simulink model "gm_ThreeSines_DrSaher"  (R2018a)
settings: Solver=FixedStepDiscrete  StartTime=0.0  StopTime=0.01  RelTol=1e-3
InitFcn:
  | ST = 2e-8
  | Ts = 2e-8
libraries: hdlmdlgenlib x97, hdlsllib x13, simulink x7, powerlib x1
(part 1 of 3)
settings Model: SimulationMode=accelerator  Creator=aaala  LastModifiedBy=aaala
settings OptimizationCC: BlockReduction=off  ConditionallyExecuteInputs=off  DefaultParameterBehavior=Inlined
settings DebuggingCC: AlgebraicLoopMsg=error  InheritedTsInSrcMsg=none  SingleTaskRateTransMsg=error
settings HardwareCC: ProdBitPerPointer=32  ProdBitPerSizeT=32  ProdBitPerPtrDiffT=32  ProdLargestAtomicFloat=None  ProdIntDivRoundTo=Undefined  ProdEndianess=Unspecified  ProdWordSize=32  ProdHWDeviceType=ASIC/FPGA->ASIC/FPGA  TargetBitPerPointer=64  TargetBitPerSizeT=64  TargetBitPerPtrDiffT=64  TargetLongLongMode=on  TargetIntDivRoundTo=Zero  TargetEndianess=LittleEndian  TargetWordSize=64  TargetHWDeviceType=Custom Processor->MATLAB Host Computer  ProdEqTarget=off

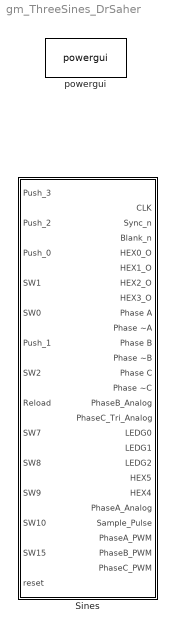
== system gm_ThreeSines_DrSaher ==
  "Sines " : Subsystem
  powergui : powerlib/powergui  Priority=1  SimulationMode=Discrete  SampleTime=ST  frequency=60  Iterations=50  frequencyindice=60  Pbase=100e6  ErrMax=1e-4  UnitsV=kV  UnitsW=MW  buscounter=0  FunctionMessages=off  echomessages=off  EnableUseOfTLC=off  CurrentSourceSwitches=off  DisableSnubberDevices=off  DisableRonSwitches=off  DisableVfSwitches=off  DisplayEquations=off  SolverType=Tustin/Backward Euler (TBE)  Interpol=off  ExternalGateDelay=off  methode=off  Ts=100  x0status=blocks  SPID=on  SwTol=0  HookPort=off  RestoreLinks=warning  ResistiveCurrentMeasurement=off  Frange=[0:2:500]  Ylog=off  Xlog=on  ShowGrid=off  save=off  variable=ZData  structure=0  ZoomFFT=off  StartTime=0.0  cycles=1  DisplayStyle=1  fundamental=60  FreqAxis=off  MaxFrequency=1000  frequencyindicesteady=1  RmsSteady=1  display=off

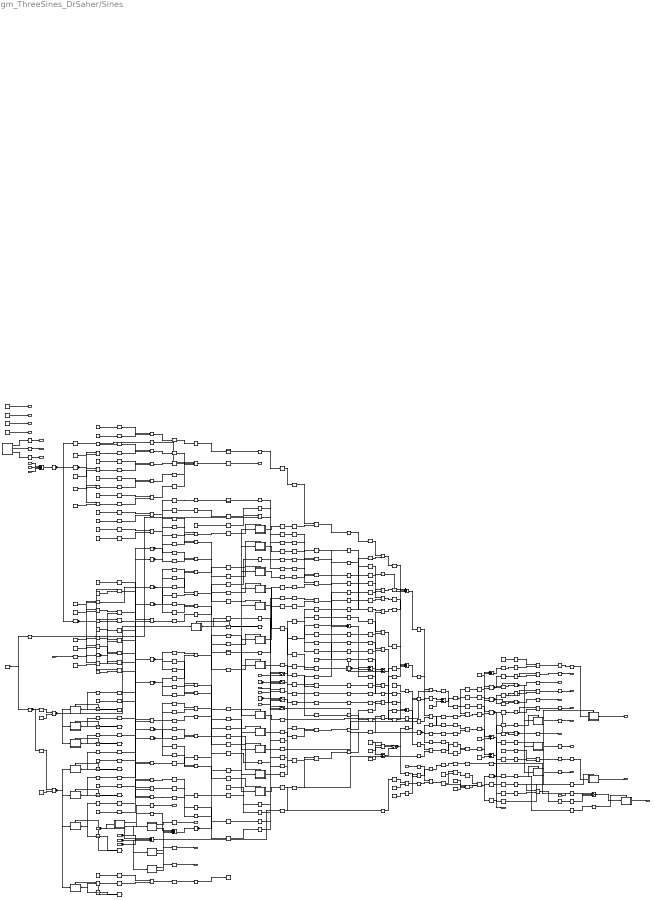
== system gm_ThreeSines_DrSaher/Sines  ==
  note: 999945
  "Push_3 " : Inport  OutDataTypeStr=boolean  PortDimensions=1  SampleTime=2e-08
  Push_2 : Inport  Port=2  OutDataTypeStr=boolean  PortDimensions=1  SampleTime=2e-08
  Push_0 : Inport  Port=3  OutDataTypeStr=boolean  PortDimensions=1  SampleTime=2e-08
  SW1 : Inport  Port=4  OutDataTypeStr=boolean  PortDimensions=1  SampleTime=2e-08
  SW0 : Inport  Port=5  OutDataTypeStr=boolean  PortDimensions=1  SampleTime=2e-08
  Push_1 : Inport  Port=6  OutDataTypeStr=boolean  PortDimensions=1  SampleTime=2e-08
  "SW2 " : Inport  Port=7  OutDataTypeStr=boolean  PortDimensions=1  SampleTime=2e-08
  Reload : Inport  Port=8  OutDataTypeStr=boolean  PortDimensions=1  SampleTime=2e-08
  "SW7 " : Inport  Port=9  OutDataTypeStr=boolean  PortDimensions=1  SampleTime=2e-08
  SW8 : Inport  Port=10  OutDataTypeStr=boolean  PortDimensions=1  SampleTime=2e-08
  SW9 : Inport  Port=11  OutDataTypeStr=boolean  PortDimensions=1  SampleTime=2e-08
  SW10 : Inport  Port=12  OutDataTypeStr=boolean  PortDimensions=1  SampleTime=2e-08
  SW15 : Inport  Port=13  OutDataTypeStr=boolean  PortDimensions=1  SampleTime=2e-08
  reset : Inport  Port=14  OutDataTypeStr=boolean  PortDimensions=1  SampleTime=2e-08
  Constant : Constant  Value=fi(0,0,32,0,'hex','00001387')  OutDataTypeStr=uint32  SampleTime=-1
  Constant10 : Constant  Value=fi(0,1,16,11,'hex','6000')  OutDataTypeStr=fixdt(1, 16, 11)  SampleTime=-1
  Constant11 : Constant  Value=fi(0,1,16,13,'hex','2000')  OutDataTypeStr=fixdt(1, 16, 13)  SampleTime=-1
  Constant12 : Constant  Value=fi(0,1,16,3,'hex','4d20')  OutDataTypeStr=fixdt(1, 16, 3)  SampleTime=-1
  Constant13 : Constant  Value=fi(0,0,20,0,'hex','51603')  OutDataTypeStr=fixdt(0, 20, 0)  SampleTime=-1
  Constant14 : Constant  Value=fi(0,1,16,6,'hex','6540')  OutDataTypeStr=fixdt(1, 16, 6)  SampleTime=-1
  Constant15 : Constant  Value=fi(0,0,3,0,'hex','4')  OutDataTypeStr=fixdt(0, 3, 0)  SampleTime=-1
  Constant17 : Constant  Value=fi(0,0,20,0,'hex','a2c06')  OutDataTypeStr=fixdt(0, 20, 0)  SampleTime=-1
  Constant22 : Constant  Value=fi(0,0,1,0,'hex','1')  OutDataTypeStr=boolean  SampleTime=-1
  Constant23 : Constant  Value=fi(0,0,1,0,'hex','1')  OutDataTypeStr=boolean  SampleTime=-1
  Constant24 : Constant  Value=fi(0,0,1,0,'hex','1')  OutDataTypeStr=boolean  SampleTime=-1
  Constant25 : Constant  Value=fi(0,1,16,11,'hex','6000')  OutDataTypeStr=fixdt(1, 16, 11)  SampleTime=-1
  Constant{26,30,33,35,79} (5 alike) : Constant  Value=fi(0,1,16,14,'hex','4000')  OutDataTypeStr=fixdt(1, 16, 14)  SampleTime=-1
  Constant27 : Constant  Value=fi(0,1,16,11,'hex','6000')  OutDataTypeStr=fixdt(1, 16, 11)  SampleTime=-1
  Constant28 : Constant  Value=fi(0,1,16,10,'hex','0000')  OutDataTypeStr=fixdt(1, 16, 10)  SampleTime=-1
  Constant31 : Constant  Value=fi(0,1,16,15,'hex','8000')  OutDataTypeStr=fixdt(1, 16, 15)  SampleTime=-1
  Constant34 : Constant  Value=fi(0,1,16,10,'hex','0000')  OutDataTypeStr=fixdt(1, 16, 10)  SampleTime=-1
  Constant36 : Constant  Value=fi(0,1,16,13,'hex','4000')  OutDataTypeStr=fixdt(1, 16, 13)  SampleTime=-1
  Constant37 : Constant  Value=fi(0,1,16,13,'hex','6000')  OutDataTypeStr=fixdt(1, 16, 13)  SampleTime=-1
  Constant38 : Constant  Value=fi(0,1,16,13,'hex','4000')  OutDataTypeStr=fixdt(1, 16, 13)  SampleTime=-1
  Constant39 : Constant  Value=fi(0,1,16,13,'hex','6000')  OutDataTypeStr=fixdt(1, 16, 13)  SampleTime=-1
  Constant4 : Constant  Value=fi(0,0,32,0,'hex','000009c3')  OutDataTypeStr=uint32  SampleTime=-1
  Constant78 : Constant  Value=fi(0,1,16,10,'hex','0000')  OutDataTypeStr=fixdt(1, 16, 10)  SampleTime=-1
  Constant80 : Constant  Value=fi(0,1,16,13,'hex','4000')  OutDataTypeStr=fixdt(1, 16, 13)  SampleTime=-1
  Constant81 : Constant  Value=fi(0,1,16,13,'hex','6000')  OutDataTypeStr=fixdt(1, 16, 13)  SampleTime=-1
  Constant82 : Constant  Value=fi(0,0,7,0,'hex','40')  OutDataTypeStr=fixdt(0, 7, 0)  SampleTime=-1
  Constant83 : Constant  Value=fi(0,0,7,0,'hex','79')  OutDataTypeStr=fixdt(0, 7, 0)  SampleTime=-1
  Constant84 : Constant  Value=fi(0,0,7,0,'hex','24')  OutDataTypeStr=fixdt(0, 7, 0)  SampleTime=-1
  Constant85 : Constant  Value=fi(0,0,7,0,'hex','30')  OutDataTypeStr=fixdt(0, 7, 0)  SampleTime=-1
  Counter Limited : simulink/Sources/Counter Limited  uplimit=double(4999)  tsamp=2e-08
  Counter Limited1 : simulink/Sources/Counter Limited  uplimit=double(4114)  tsamp=2e-08
  DAC Control : Subsystem
  Data Type Conversion{,3,27..28} (4 alike) : DataTypeConversion  OutDataTypeStr=fixdt(0, 10, 0)  SampleTime=2e-08
  Data Type Conversion1 : DataTypeConversion  OutDataTypeStr=fixdt(1, 16, 10)  SampleTime=2e-08
  Data Type Conversion{9,11,13,15,18,20,22,24,29..30,33,36} (12 alike) : DataTypeConversion  OutDataTypeStr=fixdt(1, 16, 12)  SampleTime=2e-08
  Data Type Conversion25 : DataTypeConversion  OutDataTypeStr=fixdt(1, 16, 10)  SampleTime=2e-08
  Data Type Conversion26 : DataTypeConversion  OutDataTypeStr=fixdt(1, 16, 10)  SampleTime=2e-08
  Delay{,1..5} (6 alike) : Delay  DelayLength=double(100)  InitialCondition=0  InputProcessing=Inherited  SampleTime=2e-08
  From{,1..57,59..65,80} (66 alike) : hdlmdlgenlib/Buffer
      settings: SourceProductName=HDL Coder  SourceProductBaseCode=HD
  Gain : Product  Inputs=**  OutDataTypeStr=fixdt(1, 66, 33)  SampleTime=2e-08
  Gain1 : Product  Inputs=**  OutDataTypeStr=fixdt(1, 32, 19)  SampleTime=2e-08
  Gain11 : Product  Inputs=**  OutDataTypeStr=fixdt(0, 48, 38)  SampleTime=2e-08
  Gain11_const : Constant  Value=fi(0,0,24,38,'hex','ed3038')  OutDataTypeStr=fixdt(0, 24, 38)  SampleTime=-1
  Gain13 : Product  Inputs=**  OutDataTypeStr=fixdt(0, 48, 39)  SampleTime=2e-08
  Gain13_const : Constant  Value=fi(0,0,24,39,'hex','9e2025')  OutDataTypeStr=fixdt(0, 24, 39)  SampleTime=-1
  Gain15 : Product  Inputs=**  OutDataTypeStr=fixdt(0, 48, 41)  SampleTime=2e-08
  Gain15_const : Constant  Value=fi(0,0,24,41,'hex','d2d587')  OutDataTypeStr=fixdt(0, 24, 41)  SampleTime=-1
  Gain18 : Product  Inputs=**  OutDataTypeStr=fixdt(0, 48, 38)  SampleTime=2e-08
  Gain18_const : Constant  Value=fi(0,0,24,38,'hex','ed3038')  OutDataTypeStr=fixdt(0, 24, 38)  SampleTime=-1
  Gain1_const : Constant  Value=fi(0,1,16,9,'hex','5540')  OutDataTypeStr=fixdt(1, 16, 9)  SampleTime=-1
  Gain20 : Product  Inputs=**  OutDataTypeStr=fixdt(0, 48, 39)  SampleTime=2e-08
  Gain20_const : Constant  Value=fi(0,0,24,39,'hex','9e2025')  OutDataTypeStr=fixdt(0, 24, 39)  SampleTime=-1
  Gain22 : Product  Inputs=**  OutDataTypeStr=fixdt(0, 48, 41)  SampleTime=2e-08
  Gain22_const : Constant  Value=fi(0,0,24,41,'hex','d2d587')  OutDataTypeStr=fixdt(0, 24, 41)  SampleTime=-1
  Gain24 : Product  Inputs=**  OutDataTypeStr=fixdt(0, 48, 37)  SampleTime=2e-08
  Gain24_const : Constant  Value=fi(0,0,24,37,'hex','c5a82f')  OutDataTypeStr=fixdt(0, 24, 37)  SampleTime=-1
  Gain25 : Product  Inputs=**  OutDataTypeStr=fixdt(1, 66, 42)  SampleTime=2e-08
  Gain25_const : Constant  Value=fi(0,1,33,42,'hex','0d1b71759')  OutDataTypeStr=fixdt(1, 33, 42)  SampleTime=-1
  Gain26 : Product  Inputs=**  OutDataTypeStr=fixdt(1, 32, 19)  SampleTime=2e-08
  Gain26_const : Constant  Value=fi(0,1,16,9,'hex','5540')  OutDataTypeStr=fixdt(1, 16, 9)  SampleTime=-1
  Gain27 : Product  Inputs=**  OutDataTypeStr=fixdt(1, 32, 19)  SampleTime=2e-08
  Gain27_const : Constant  Value=fi(0,1,16,9,'hex','5540')  OutDataTypeStr=fixdt(1, 16, 9)  SampleTime=-1
  Gain31 : Product  Inputs=**  OutDataTypeStr=fixdt(0, 48, 37)  SampleTime=2e-08
  Gain31_const : Constant  Value=fi(0,0,24,37,'hex','c5a82f')  OutDataTypeStr=fixdt(0, 24, 37)  SampleTime=-1
  Gain32 : Product  Inputs=**  OutDataTypeStr=fixdt(0, 48, 38)  SampleTime=2e-08
  Gain32_const : Constant  Value=fi(0,0,24,38,'hex','ed3038')  OutDataTypeStr=fixdt(0, 24, 38)  SampleTime=-1
  Gain33 : Product  Inputs=**  OutDataTypeStr=fixdt(0, 48, 39)  SampleTime=2e-08
  Gain33_const : Constant  Value=fi(0,0,24,39,'hex','9e2025')  OutDataTypeStr=fixdt(0, 24, 39)  SampleTime=-1
  Gain34 : Product  Inputs=**  OutDataTypeStr=fixdt(0, 48, 41)  SampleTime=2e-08
  Gain34_const : Constant  Value=fi(0,0,24,41,'hex','d2d587')  OutDataTypeStr=fixdt(0, 24, 41)  SampleTime=-1
  Gain9 : Product  Inputs=**  OutDataTypeStr=fixdt(0, 48, 37)  SampleTime=2e-08
  Gain9_const : Constant  Value=fi(0,0,24,37,'hex','c5a82f')  OutDataTypeStr=fixdt(0, 24, 37)  SampleTime=-1
  Gain_const : Constant  Value=fi(0,1,33,33,'hex','0d1981ff6')  OutDataTypeStr=fixdt(1, 33, 33)  SampleTime=-1
  Goto{,1,3..16,18..21,35..36,41..49} (31 alike) : hdlmdlgenlib/Buffer
      settings: SourceProductName=HDL Coder  SourceProductBaseCode=HD
  H : Constant  Value=fi(0,0,7,0,'hex','09')  OutDataTypeStr=fixdt(0, 7, 0)  SampleTime=-1
  HDL Counter : hdlsllib/Sources/HDL Counter  CountType=Count limited  CountInit=double(1)  CountStep=double(1)  CountMax=double(66663)  CountFromType=Initial value  CountFrom=double(1)  CountResetPort=off  CountLoadPort=off  CountEnbPort=on  CountDirPort=off  CountDataType=Unsigned  CountWordLen=24  CountFracLen=0  CountSampTime=2e-08
      settings: SourceProductBaseCode=HD
  HDL Counter1 : hdlsllib/Sources/HDL Counter  CountType=Count limited  CountInit=double(1)  CountStep=double(1)  CountMax=double(111105)  CountFromType=Initial value  CountFrom=double(1)  CountResetPort=off  CountLoadPort=off  CountEnbPort=on  CountDirPort=off  CountDataType=Unsigned  CountWordLen=24  CountFracLen=0  CountSampTime=2e-08
      settings: SourceProductBaseCode=HD
  HDL Counter10 : hdlsllib/Sources/HDL Counter  CountType=Count limited  CountInit=double(1)  CountStep=double(1)  CountMax=double(333315)  CountFromType=Initial value  CountFrom=double(1)  CountResetPort=off  CountLoadPort=off  CountEnbPort=off  CountDirPort=off  CountDataType=Unsigned  CountWordLen=24  CountFracLen=0  CountSampTime=2e-08
      settings: SourceProductBaseCode=HD
  HDL Counter11 : hdlsllib/Sources/HDL Counter  CountType=Count limited  CountInit=double(1)  CountStep=double(1)  CountMax=double(999945)  CountFromType=Initial value  CountFrom=double(1)  CountResetPort=off  CountLoadPort=off  CountEnbPort=off  CountDirPort=off  CountDataType=Unsigned  CountWordLen=24  CountFracLen=0  CountSampTime=2e-08
      settings: SourceProductBaseCode=HD
  HDL Counter12 : hdlsllib/Sources/HDL Counter  CountType=Count limited  CountInit=double(1)  CountStep=double(1)  CountMax=double(405)  CountFromType=Initial value  CountFrom=double(1)  CountResetPort=on  CountLoadPort=off  CountEnbPort=on  CountDirPort=off  CountDataType=Unsigned  CountWordLen=9  CountFracLen=0  CountSampTime=2e-08
      settings: SourceProductBaseCode=HD
  HDL Counter2 : hdlsllib/Sources/HDL Counter  CountType=Count limited  CountInit=double(1)  CountStep=double(1)  CountMax=double(333315)  CountFromType=Initial value  CountFrom=double(1)  CountResetPort=off  CountLoadPort=off  CountEnbPort=on  CountDirPort=off  CountDataType=Unsigned  CountWordLen=24  CountFracLen=0  CountSampTime=2e-08
      settings: SourceProductBaseCode=HD
  HDL Counter3 : hdlsllib/Sources/HDL Counter  CountType=Count limited  CountInit=double(0)  CountStep=double(1)  CountMax=double(999945)  CountFromType=Initial value  CountFrom=double(0)  CountResetPort=off  CountLoadPort=off  CountEnbPort=on  CountDirPort=off  CountDataType=Unsigned  CountWordLen=24  CountFracLen=0  CountSampTime=2e-08
      settings: SourceProductBaseCode=HD
  HDL Counter4 : hdlsllib/Sources/HDL Counter  CountType=Count limited  CountInit=double(1)  CountStep=double(1)  CountMax=double(66663)  CountFromType=Initial value  CountFrom=double(1)  CountResetPort=off  CountLoadPort=off  CountEnbPort=on  CountDirPort=off  CountDataType=Unsigned  CountWordLen=24  CountFracLen=0  CountSampTime=2e-08
      settings: SourceProductBaseCode=HD
  HDL Counter5 : hdlsllib/Sources/HDL Counter  CountType=Count limited  CountInit=double(1)  CountStep=double(1)  CountMax=double(111105)  CountFromType=Initial value  CountFrom=double(1)  CountResetPort=off  CountLoadPort=off  CountEnbPort=on  CountDirPort=off  CountDataType=Unsigned  CountWordLen=24  CountFracLen=0  CountSampTime=2e-08
      settings: SourceProductBaseCode=HD
  HDL Counter6 : hdlsllib/Sources/HDL Counter  CountType=Count limited  CountInit=double(1)  CountStep=double(1)  CountMax=double(333315)  CountFromType=Initial value  CountFrom=double(1)  CountResetPort=off  CountLoadPort=off  CountEnbPort=on  CountDirPort=off  CountDataType=Unsigned  CountWordLen=24  CountFracLen=0  CountSampTime=2e-08
      settings: SourceProductBaseCode=HD
  HDL Counter7 : hdlsllib/Sources/HDL Counter  CountType=Count limited  CountInit=double(1)  CountStep=double(1)  CountMax=double(999945)  CountFromType=Initial value  CountFrom=double(1)  CountResetPort=off  CountLoadPort=off  CountEnbPort=on  CountDirPort=off  CountDataType=Unsigned  CountWordLen=24  CountFracLen=0  CountSampTime=2e-08
      settings: SourceProductBaseCode=HD
  HDL Counter8 : hdlsllib/Sources/HDL Counter  CountType=Count limited  CountInit=double(1)  CountStep=double(1)  CountMax=double(66663)  CountFromType=Initial value  CountFrom=double(1)  CountResetPort=off  CountLoadPort=off  CountEnbPort=off  CountDirPort=off  CountDataType=Unsigned  CountWordLen=24  CountFracLen=0  CountSampTime=2e-08
      settings: SourceProductBaseCode=HD
  HDL Counter9 : hdlsllib/Sources/HDL Counter  CountType=Count limited  CountInit=double(1)  CountStep=double(1)  CountMax=double(111105)  CountFromType=Initial value  CountFrom=double(1)  CountResetPort=off  CountLoadPort=off  CountEnbPort=off  CountDirPort=off  CountDataType=Unsigned  CountWordLen=24  CountFracLen=0  CountSampTime=2e-08
      settings: SourceProductBaseCode=HD
  HEX0 : Subsystem
  HEX1 : Subsystem
  HEX2 : Subsystem
  HEX3 : Subsystem
  HwModeRegister{,1..89} (90 alike) : Delay  DelayLength=double(1)  InitialCondition=0  InputProcessing=Inherited  SampleTime=2e-08
  Logical Operator{,1..7,9,25..26,28..29,52} (14 alike) : Logic  Operator=NOT  Inputs=1  AllPortsSameDT=off  OutDataTypeStr=boolean  SampleTime=2e-08
  Logical Operator{8,10..24,27,38,41..42,45,49,51} (23 alike) : Logic  AllPortsSameDT=off  OutDataTypeStr=boolean  SampleTime=2e-08
  Logical Operator34 : Logic  Operator=OR  AllPortsSameDT=off  OutDataTypeStr=boolean  SampleTime=2e-08
  Multiply{,1..2,8,14..16,22..23} (9 alike) : Product  Inputs=**  OutDataTypeStr=fixdt(1, 38, 29)  SampleTime=2e-08
  Multiply10 : Product  Inputs=**  OutDataTypeStr=fixdt(1, 94, 72)  SampleTime=2e-08
  Multiply{5..7,11..13,19..21} (9 alike) : Product  Inputs=**  OutDataTypeStr=fixdt(1, 54, 43)  SampleTime=2e-08
  Multiply17 : Product  Inputs=**  OutDataTypeStr=fixdt(1, 78, 58)  SampleTime=2e-08
  Multiply18 : Product  Inputs=**  OutDataTypeStr=fixdt(1, 94, 72)  SampleTime=2e-08
  Multiply{27..30} (4 alike) : Product  Inputs=**  OutDataTypeStr=fixdt(0, 7, 0)  SampleTime=2e-08
  Multiply3 : Product  Inputs=**  OutDataTypeStr=fixdt(1, 78, 58)  SampleTime=2e-08
  Multiply4 : Product  Inputs=**  OutDataTypeStr=fixdt(1, 94, 72)  SampleTime=2e-08
  Multiply9 : Product  Inputs=**  OutDataTypeStr=fixdt(1, 78, 58)  SampleTime=2e-08
  Multiport Switch1 : MultiPortSwitch  DataPortOrder=Zero-based contiguous  Inputs=4  DiagnosticForDefault=None  zeroidx=on  OutDataTypeStr=fixdt(0, 7, 0)  SampleTime=2e-08
  Phase A PWM : RelationalOperator  OutDataTypeStr=boolean  SampleTime=2e-08  RndMeth=Nearest
  Phase B PWM : RelationalOperator  OutDataTypeStr=boolean  SampleTime=2e-08  RndMeth=Nearest
  Phase C PWM : RelationalOperator  OutDataTypeStr=boolean  SampleTime=2e-08  RndMeth=Nearest
  PipelineRegister{,1..44} (45 alike) : Delay  DelayLength=double(1)  InitialCondition=0  InputProcessing=Inherited  SampleTime=2e-08
  Relational Operator : RelationalOperator  Operator=<  OutDataTypeStr=boolean  SampleTime=2e-08  RndMeth=Nearest
  Relational Operator{1..3,12..18,20,34..37} (15 alike) : RelationalOperator  Operator===  OutDataTypeStr=boolean  SampleTime=2e-08  RndMeth=Nearest
  Relational Operator4 : RelationalOperator  OutDataTypeStr=boolean  SampleTime=2e-08  RndMeth=Nearest
  Relational Operator8 : RelationalOperator  OutDataTypeStr=boolean  SampleTime=2e-08  RndMeth=Nearest
  Sin10 : Subsystem
  Sin11 : Subsystem
  Sin12 : Subsystem
  Sin13 : Subsystem
  Sin14 : Subsystem
  Sin15 : Subsystem
  Sin4 : Subsystem
  Sin5 : Subsystem
  Sin6 : Subsystem
  Sin7 : Subsystem
  Sin8 : Subsystem
  Sin9 : Subsystem
  Subsystem : Subsystem
  Subsystem1 : Subsystem
  Subsystem10 : Subsystem
  Subsystem11 : Subsystem
  Subsystem12 : Subsystem
  Subsystem13 : Subsystem
  Subsystem2 : Subsystem
  Subsystem3 : Subsystem
  Subsystem4 : Subsystem
  Subsystem5 : Subsystem
  Subsystem6 : Subsystem
  Subsystem7 : Subsystem
  Subsystem8 : Subsystem
  Subsystem9 : Subsystem
  Sum : Sum  Inputs=-+  AccumDataTypeStr=fixdt(1, 33, 0)  OutDataTypeStr=fixdt(1, 33, 0)  SampleTime=2e-08
  Sum13 : Sum  AccumDataTypeStr=fixdt(1, 95, 72)  OutDataTypeStr=fixdt(1, 95, 72)  SampleTime=2e-08
  Sum14 : Sum  Inputs=++++  AccumDataTypeStr=fixdt(1, 22, 15)  OutDataTypeStr=fixdt(1, 22, 15)  SampleTime=2e-08
  Sum15 : Sum  Inputs=+++  AccumDataTypeStr=fixdt(0, 10, 0)  OutDataTypeStr=fixdt(0, 10, 0)  SampleTime=2e-08
  Sum16 : Sum  Inputs=+-  AccumDataTypeStr=fixdt(1, 67, 42)  OutDataTypeStr=fixdt(1, 67, 42)  SampleTime=2e-08
  Sum17 : Sum  AccumDataTypeStr=fixdt(1, 95, 72)  OutDataTypeStr=fixdt(1, 95, 72)  SampleTime=2e-08
  Sum18 : Sum  AccumDataTypeStr=fixdt(1, 95, 72)  OutDataTypeStr=fixdt(1, 95, 72)  SampleTime=2e-08
  Sum19 : Sum  Inputs=++++  AccumDataTypeStr=fixdt(1, 56, 43)  OutDataTypeStr=fixdt(1, 56, 43)  SampleTime=2e-08
  Sum20 : Sum  Inputs=++++  AccumDataTypeStr=fixdt(1, 56, 43)  OutDataTypeStr=fixdt(1, 56, 43)  SampleTime=2e-08
  Sum21_stage2 : Sum  Inputs=-+  AccumDataTypeStr=fixdt(1, 18, 14)  OutDataTypeStr=fixdt(1, 18, 14)  SampleTime=2e-08
  Sum21_stage3 : Sum  Inputs=+-  AccumDataTypeStr=fixdt(1, 18, 14)  OutDataTypeStr=fixdt(1, 18, 14)  SampleTime=2e-08
  Sum22 : Sum  Inputs=++++  AccumDataTypeStr=fixdt(1, 56, 43)  OutDataTypeStr=fixdt(1, 56, 43)  SampleTime=2e-08
  Sum23 : Sum  Inputs=+-  AccumDataTypeStr=fixdt(1, 19, 14)  OutDataTypeStr=fixdt(1, 19, 14)  SampleTime=2e-08
  Sum24 : Sum  Inputs=++++  AccumDataTypeStr=fixdt(0, 10, 0)  OutDataTypeStr=fixdt(0, 10, 0)  SampleTime=2e-08
  Switch : Switch  Criteria=u2 > Threshold  Threshold=double(0)  OutDataTypeStr=fixdt(1, 33, 0)  SampleTime=2e-08
  Switch{1..4} (4 alike) : Switch  Criteria=u2 > Threshold  Threshold=double(0)  OutDataTypeStr=fixdt(1, 16, 14)  SampleTime=2e-08
  Switch13 : Switch  Criteria=u2 > Threshold  Threshold=double(0)  OutDataTypeStr=fixdt(0, 10, 0)  SampleTime=2e-08
  Unit Delay{,1..7} (8 alike) : UnitDelay  SampleTime=2e-08
  aPA_Save : Subsystem
  aPB_Save : Subsystem
  aPC_Save : Subsystem
  bPA_Save : Subsystem
  bPB_Save : Subsystem
  bPC_Save : Subsystem
  cPA_Save : Subsystem
  cPB_Save : Subsystem
  cPC_Save : Subsystem
  dPA_Save : Subsystem
  dPB_Save : Subsystem
  dPC_Save : Subsystem
  delayMatch{,47,59..64,67..69} (11 alike) : Delay  DelayLength=double(2)  InitialCondition=0  InputProcessing=Inherited  SampleTime=2e-08
  delayMatch{1,4,7,10..11,15,18,21,24..25,29,32,35,38..39} (15 alike) : Delay  DelayLength=double(4)  InitialCondition=0  InputProcessing=Inherited  SampleTime=2e-08
  delayMatch12 : Delay  DelayLength=double(14)  InitialCondition=0  InputProcessing=Inherited  SampleTime=2e-08
  delayMatch{13..14,27..28,41..42} (6 alike) : Delay  DelayLength=double(20)  InitialCondition=0  InputProcessing=Inherited  SampleTime=2e-08
  delayMatch{2,5,8,16,19,22,30,33,36} (9 alike) : Delay  DelayLength=double(10)  InitialCondition=0  InputProcessing=Inherited  SampleTime=2e-08
  delayMatch{3,6,9,17,20,23,31,34,37} (9 alike) : Delay  DelayLength=double(16)  InitialCondition=0  InputProcessing=Inherited  SampleTime=2e-08
  delayMatch26 : Delay  DelayLength=double(14)  InitialCondition=0  InputProcessing=Inherited  SampleTime=2e-08
  delayMatch40 : Delay  DelayLength=double(14)  InitialCondition=0  InputProcessing=Inherited  SampleTime=2e-08
  delayMatch{43,45..46,48,52..58,66} (12 alike) : Delay  DelayLength=double(24)  InitialCondition=0  InputProcessing=Inherited  SampleTime=2e-08
  delayMatch{44,49..51,65} (5 alike) : Delay  DelayLength=double(22)  InitialCondition=0  InputProcessing=Inherited  SampleTime=2e-08
  "CLK " : Outport  OutDataTypeStr=boolean
  Sync_n : Outport  Port=2
  Blank_n : Outport  Port=3
  HEX0_O : Outport  Port=4
  HEX1_O : Outport  Port=5
  HEX2_O : Outport  Port=6
  HEX3_O : Outport  Port=7
  Phase A : Outport  Port=8
  Phase ~A : Outport  Port=9
  Phase B : Outport  Port=10
  Phase ~B : Outport  Port=11
  Phase C : Outport  Port=12
  Phase ~C : Outport  Port=13
  PhaseB_Analog : Outport  Port=14
  PhaseC_Tri_Analog : Outport  Port=15
  LEDG0 : Outport  Port=16
  LEDG1 : Outport  Port=17
  LEDG2 : Outport  Port=18
  HEX5 : Outport  Port=19
  HEX4 : Outport  Port=20
  PhaseA_Analog : Outport  Port=21
  Sample_Pulse : Outport  Port=22
  PhaseA_PWM : Outport  Port=23
  PhaseB_PWM : Outport  Port=24
  PhaseC_PWM : Outport  Port=25
  wires:
  "Push_3 "/1 -> Sum24/1, HEX3/1(Push_3)
  Push_2/1 -> Sum24/2, HEX2/1(Push_2)
  Push_0/1 -> Sum24/4, HEX0/1(Push_0)
  SW1/1 -> Sum15/2
  SW0/1 -> Sum15/1
  Push_1/1 -> Sum24/3, HEX1/1(Push_1)
  "SW2 "/1 -> Sum15/3
  Reload/1 -> Goto36/1
  "SW7 "/1 -> Switch1/2
  SW8/1 -> Switch2/2
  SW9/1 -> Switch3/2
  SW10/1 -> Switch4/2
  delayMatch45/1 -> Switch13/2
  reset/1 -> Logical Operator28/1
  Constant/1 -> Sum/2
  Constant10/1 -> Sum13/2
  Constant11/1 -> Sum23/2, Sum21_stage2/2
  Constant12/1 -> Relational Operator1/2
  Constant13/1 -> Relational Operator4/2
  Constant14/1 -> Relational Operator2/2
  Constant15/1 -> Relational Operator3/2
  Constant17/1 -> Relational Operator8/2
  Constant22/1 -> LEDG0/1
  Constant23/1 -> LEDG1/1
  Constant24/1 -> LEDG2/1
  Constant25/1 -> Sum18/2
  Constant26/1 -> Sum16/2
  Constant27/1 -> Sum17/2
  Constant28/1 -> Relational Operator18/2
  Constant30/1 -> Switch4/3, Switch3/3, Switch2/3, Switch1/3
  Constant31/1 -> Switch4/1, Switch3/1, Switch2/1, Switch1/1
  Constant33/1 -> Relational Operator12/2
  Constant34/1 -> Relational Operator20/2
  Constant35/1 -> Relational Operator13/2
  Constant36/1 -> Relational Operator14/2
  Constant37/1 -> Relational Operator15/2
  Constant38/1 -> Relational Operator16/2
  Constant39/1 -> Relational Operator17/2
  Constant4/1 -> Relational Operator/2
  Constant78/1 -> Relational Operator34/2
  Constant79/1 -> Relational Operator35/2
  Constant80/1 -> Relational Operator36/2
  Constant81/1 -> Relational Operator37/2
  Constant82/1 -> HwModeRegister34/1
  Constant83/1 -> HwModeRegister36/1
  Constant84/1 -> HwModeRegister38/1
  Constant85/1 -> HwModeRegister42/1
  Counter Limited/1 -> Switch/1, Sum/1, Relational Operator/1
  Counter Limited1/1 -> Relational Operator1/1
  delayMatch52/1 -> "CLK "/1
  delayMatch53/1 -> Sync_n/1
  delayMatch54/1 -> Blank_n/1
  Data Type Conversion/1 -> Goto35/1
  Data Type Conversion1/1 -> HwModeRegister59/1
  Data Type Conversion11/1 -> Sin5/1(In1)
  Data Type Conversion13/1 -> Sin6/1(In1)
  Data Type Conversion15/1 -> Sin7/1(In1)
  Data Type Conversion18/1 -> Sin9/1(In1)
  Data Type Conversion20/1 -> Sin10/1(In1)
  Data Type Conversion22/1 -> Sin11/1(In1)
  Data Type Conversion24/1 -> Sin8/1(In1)
  Data Type Conversion25/1 -> HwModeRegister77/1
  Data Type Conversion26/1 -> HwModeRegister79/1
  Data Type Conversion27/1 -> Switch13/3
  Data Type Conversion28/1 -> Subsystem8/1(In1)
  Data Type Conversion29/1 -> Sin12/1(In1)
  Data Type Conversion3/1 -> Subsystem9/1(In1)
  Data Type Conversion30/1 -> Sin13/1(In1)
  Data Type Conversion33/1 -> Sin14/1(In1)
  Data Type Conversion36/1 -> Sin15/1(In1)
  Data Type Conversion9/1 -> Sin4/1(In1)
  Delay/1 -> Logical Operator8/2
  Delay1/1 -> Logical Operator10/2
  Delay2/1 -> Logical Operator24/2
  Delay3/1 -> Logical Operator18/2
  Delay4/1 -> Logical Operator51/2
  Delay5/1 -> Logical Operator38/2
  From/1 -> HwModeRegister12/1
  From1/1 -> Logical Operator22/2
  From10/1 -> HwModeRegister24/1
  delayMatch10/1 -> Sum19/4
  From12/1 -> Logical Operator45/2
  From13/1 -> Logical Operator42/2
  From14/1 -> HwModeRegister52/1
  From15/1 -> Relational Operator20/1, Relational Operator18/1, Relational Operator17/1, Relational Operator16/1, Relational Operator15/1, Relational Operator14/1, Relational Operator13/1, Relational Operator12/1
  From16/1 -> dPA_Save/1(MulNumber), aPA_Save/1(MulNumber), bPA_Save/1(MulNumber), cPA_Save/1(MulNumber)
  delayMatch14/1 -> Phase A PWM/1
  delayMatch49/1 -> Subsystem11/Enable
  delayMatch13/1 -> HwModeRegister45/1
  From2/1 -> Logical Operator20/2
  delayMatch27/1 -> HwModeRegister5/1
  From21/1 -> dPB_Save/1(MulNumber), cPB_Save/1(MulNumber), bPB_Save/1(MulNumber), aPB_Save/1(MulNumber)
  delayMatch28/1 -> Phase B PWM/1
  From23/1 -> Logical Operator41/2
  From24/1 -> Logical Operator20/1
  From25/1 -> Logical Operator49/2
  From26/1 -> Logical Operator19/1
  From27/1 -> Logical Operator23/1
  From28/1 -> HwModeRegister30/1
  From29/1 -> Logical Operator14/1
  From3/1 -> Relational Operator4/1
  From30/1 -> HwModeRegister32/1
  From31/1 -> Relational Operator37/1, Relational Operator36/1, Relational Operator35/1, Relational Operator34/1
  From32/1 -> Logical Operator13/1
  From33/1 -> Logical Operator21/1
  From34/1 -> Logical Operator17/2
  From35/1 -> Logical Operator17/1
  From36/1 -> HwModeRegister16/1
  From37/1 -> Logical Operator14/2
  From38/1 -> Logical Operator13/2
  delayMatch47/1 -> Multiport Switch1/1
  From4/1 -> Logical Operator19/2
  From40/1 -> Logical Operator21/2
  delayMatch23/1 -> HwModeRegister11/1
  delayMatch38/1 -> Sum22/4
  From43/1 -> Logical Operator22/1
  delayMatch20/1 -> HwModeRegister9/1
  delayMatch44/1 -> Switch13/1
  delayMatch17/1 -> HwModeRegister7/1
  From47/1 -> Logical Operator16/2, Logical Operator15/2, Logical Operator12/2, Logical Operator11/2
  From48/1 -> Relational Operator3/1
  delayMatch43/1 -> Subsystem9/Enable
  From5/1 -> Logical Operator23/2
  delayMatch46/1 -> Subsystem10/Enable
  delayMatch50/1 -> Subsystem12/Enable
  delayMatch9/1 -> HwModeRegister51/1
  delayMatch41/1 -> HwModeRegister21/1
  From54/1 -> aPC_Save/1(MulNumber), bPC_Save/1(MulNumber), cPC_Save/1(MulNumber), dPC_Save/1(MulNumber)
  delayMatch6/1 -> HwModeRegister49/1
  delayMatch3/1 -> HwModeRegister47/1
  delayMatch51/1 -> Subsystem13/Enable
  delayMatch42/1 -> Phase C PWM/1
  From6/1 -> HwModeRegister14/1
  From60/1 -> Logical Operator42/1
  From61/1 -> Logical Operator41/1
  From62/1 -> Logical Operator49/1
  delayMatch37/1 -> HwModeRegister29/1
  From64/1 -> Logical Operator45/1
  delayMatch34/1 -> HwModeRegister27/1
  From7/1 -> Relational Operator8/1
  From8/1 -> HwModeRegister/1
  delayMatch31/1 -> HwModeRegister23/1
  From9/1 -> HwModeRegister2/1
  PipelineRegister28/1 -> Data Type Conversion/1
  PipelineRegister29/1 -> Data Type Conversion3/1
  PipelineRegister30/1 -> Data Type Conversion11/1
  PipelineRegister31/1 -> Data Type Conversion13/1
  PipelineRegister32/1 -> Data Type Conversion15/1
  PipelineRegister33/1 -> Data Type Conversion18/1
  PipelineRegister34/1 -> Data Type Conversion20/1
  PipelineRegister35/1 -> Data Type Conversion22/1
  PipelineRegister36/1 -> Data Type Conversion24/1
  PipelineRegister37/1 -> Sum16/1
  PipelineRegister38/1 -> Data Type Conversion28/1
  PipelineRegister39/1 -> Data Type Conversion27/1
  PipelineRegister40/1 -> Data Type Conversion29/1
  PipelineRegister41/1 -> Data Type Conversion30/1
  PipelineRegister42/1 -> Data Type Conversion33/1
  PipelineRegister43/1 -> Data Type Conversion36/1
  PipelineRegister44/1 -> Data Type Conversion9/1
  H/1 -> HEX5/1
  HDL Counter/1 -> HwModeRegister89/1
  HDL Counter1/1 -> HwModeRegister61/1
  HDL Counter10/1 -> HwModeRegister85/1
  HDL Counter11/1 -> Goto3/1, HwModeRegister87/1
  HDL Counter2/1 -> HwModeRegister63/1
  HDL Counter3/1 -> HwModeRegister65/1
  HDL Counter4/1 -> HwModeRegister73/1
  HDL Counter5/1 -> HwModeRegister67/1
  HDL Counter6/1 -> HwModeRegister69/1
  HDL Counter7/1 -> HwModeRegister71/1
  HDL Counter8/1 -> HwModeRegister81/1
  HDL Counter9/1 -> HwModeRegister83/1
  delayMatch55/1 -> HEX0_O/1
  HEX0/2(Out2) -> Sum14/4
  delayMatch56/1 -> HEX1_O/1
  HEX1/2(Out2) -> Sum14/3
  delayMatch57/1 -> HEX2_O/1
  HEX2/2(out2) -> Sum14/2
  delayMatch58/1 -> HEX3_O/1
  delayMatch/1 -> Sum14/1
  delayMatch60/1 -> Phase ~A/1
  Logical Operator11/1 -> Goto45/1
  Logical Operator12/1 -> Goto46/1
  delayMatch4/1 -> bPA_Save/Enable
  delayMatch7/1 -> cPA_Save/Enable
  Logical Operator15/1 -> Goto47/1
  Logical Operator16/1 -> Goto48/1
  delayMatch11/1 -> dPA_Save/Enable
  delayMatch62/1 -> Phase ~B/1
  delayMatch18/1 -> bPB_Save/Enable
  delayMatch21/1 -> cPB_Save/Enable
  delayMatch1/1 -> aPA_Save/Enable
  delayMatch25/1 -> dPB_Save/Enable
  delayMatch15/1 -> aPB_Save/Enable
  delayMatch61/1 -> Phase B/1
  Logical Operator25/1 -> Logical Operator18/1, Delay3/1
  delayMatch48/1 -> Subsystem8/Enable
  Logical Operator28/1 -> Logical Operator34/1
  Logical Operator29/1 -> Logical Operator34/2
  Logical Operator34/1 -> HDL Counter12/1
  delayMatch64/1 -> Phase ~C/1
  delayMatch32/1 -> bPC_Save/Enable
  delayMatch35/1 -> cPC_Save/Enable
  delayMatch39/1 -> dPC_Save/Enable
  delayMatch29/1 -> aPC_Save/Enable
  delayMatch63/1 -> Phase C/1
  Logical Operator52/1 -> Logical Operator38/1, Delay5/1
  delayMatch59/1 -> Phase A/1
  Logical Operator9/1 -> Logical Operator10/1, Delay1/1
  PipelineRegister/1 -> HwModeRegister46/1
  PipelineRegister1/1 -> HwModeRegister48/1
  PipelineRegister2/1 -> Sum13/1, Phase B PWM/2
  PipelineRegister3/1 -> Sum20/1
  PipelineRegister4/1 -> Sum20/2
  PipelineRegister5/1 -> Sum20/3
  PipelineRegister6/1 -> HwModeRegister6/1
  PipelineRegister7/1 -> HwModeRegister8/1
  PipelineRegister8/1 -> HwModeRegister28/1
  PipelineRegister9/1 -> HwModeRegister20/1
  PipelineRegister10/1 -> Sum18/1, Phase C PWM/2
  PipelineRegister11/1 -> Sum22/1
  PipelineRegister12/1 -> HwModeRegister50/1
  PipelineRegister13/1 -> Sum22/2
  PipelineRegister14/1 -> Sum22/3
  PipelineRegister15/1 -> HwModeRegister22/1
  PipelineRegister16/1 -> HwModeRegister26/1
  PipelineRegister17/1 -> Multiport Switch1/2
  PipelineRegister18/1 -> Multiport Switch1/3
  PipelineRegister19/1 -> Multiport Switch1/4
  PipelineRegister20/1 -> HwModeRegister44/1
  PipelineRegister21/1 -> Multiport Switch1/5
  PipelineRegister22/1 -> Sum17/1, Phase A PWM/2
  PipelineRegister23/1 -> Sum19/1
  PipelineRegister24/1 -> Sum19/2
  PipelineRegister25/1 -> Sum19/3
  PipelineRegister26/1 -> HwModeRegister10/1
  PipelineRegister27/1 -> HwModeRegister4/1
  delayMatch65/1 -> HEX4/1
  Phase A PWM/1 -> Logical Operator9/1, Logical Operator8/1, Delay/1
  Phase B PWM/1 -> Logical Operator25/1, Logical Operator24/1, Delay2/1
  Phase C PWM/1 -> Logical Operator52/1, Logical Operator51/1, Delay4/1
  Relational Operator/1 -> Switch/2
  Relational Operator1/1 -> Logical Operator27/2
  Relational Operator12/1 -> Logical Operator12/1
  Relational Operator13/1 -> Goto42/1
  Relational Operator14/1 -> Goto43/1
  Relational Operator15/1 -> Goto44/1
  Relational Operator16/1 -> Logical Operator15/1
  Relational Operator17/1 -> Logical Operator16/1
  Relational Operator18/1 -> Logical Operator11/1
  Relational Operator20/1 -> Goto41/1
  Relational Operator3/1 -> Logical Operator29/1
  Relational Operator34/1 -> HwModeRegister35/1
  Relational Operator35/1 -> HwModeRegister37/1
  Relational Operator36/1 -> HwModeRegister39/1
  Relational Operator37/1 -> HwModeRegister43/1
  Relational Operator4/1 -> Subsystem/1(In1), Subsystem1/1(In1), Subsystem2/1(In1), Subsystem3/1(In1)
  Relational Operator8/1 -> Subsystem7/1(In1), Subsystem4/1(In1), Subsystem5/1(In1), Subsystem6/1(In1)
  Sin10/1(Out1) -> Goto19/1
  Sin11/1(Out1) -> Sum21_stage3/2, Goto18/1
  Sin12/1(Out1) -> Goto4/1
  Sin13/1(Out1) -> Goto5/1
  Sin14/1(Out1) -> Goto6/1
  Sin15/1(Out1) -> Sum21_stage2/1, Goto7/1
  Sin4/1(Out1) -> Goto14/1
  Sin5/1(Out1) -> Goto15/1
  Sin6/1(Out1) -> Goto16/1
  Sin8/1(Out1) -> Goto21/1
  Sin9/1(Out1) -> Goto20/1
  Subsystem/1(Out1) -> HDL Counter/1, Unit Delay/1
  Subsystem1/1(Out1) -> HDL Counter1/1, Unit Delay1/1
  Subsystem10/1(Out1) -> PhaseC_Tri_Analog/1
  delayMatch67/1 -> PhaseA_PWM/1
  delayMatch68/1 -> PhaseB_PWM/1
  delayMatch69/1 -> PhaseC_PWM/1
  Subsystem2/1(Out1) -> HDL Counter2/1, Unit Delay2/1
  Subsystem3/1(Out1) -> HDL Counter3/1, Unit Delay3/1
  Subsystem4/1(Out1) -> HDL Counter4/1, Unit Delay4/1
  Subsystem5/1(Out1) -> HDL Counter5/1, Unit Delay5/1
  Subsystem6/1(Out1) -> HDL Counter6/1, Unit Delay6/1
  Subsystem7/1(Out1) -> HDL Counter7/1, Unit Delay7/1
  Subsystem8/1(Out1) -> PhaseA_Analog/1
  Subsystem9/1(Out1) -> PhaseB_Analog/1
  Sum/1 -> Switch/3
  Sum13/1 -> Data Type Conversion1/1
  Sum14/1 -> Goto12/1
  Sum15/1 -> Goto11/1
  Sum16/1 -> Goto13/1
  Sum17/1 -> Data Type Conversion25/1
  Sum18/1 -> Data Type Conversion26/1
  Sum19/1 -> HwModeRegister40/1
  Sum20/1 -> HwModeRegister54/1
  Sum21_stage3/1 -> Sum23/1
  Sum22/1 -> HwModeRegister18/1
  delayMatch24/1 -> Sum20/4
  Sum24/1 -> Goto/1
  Switch/1 -> HwModeRegister57/1, HwModeRegister75/1
  Switch1/1 -> Goto8/1
  Switch13/1 -> Subsystem10/1(In1)
  Switch2/1 -> Goto9/1
  Switch3/1 -> Goto10/1
  Switch4/1 -> Goto49/1
  delayMatch2/1 -> HwModeRegister1/1
  delayMatch16/1 -> HwModeRegister13/1
  delayMatch30/1 -> HwModeRegister31/1
  delayMatch5/1 -> HwModeRegister3/1
  delayMatch19/1 -> HwModeRegister15/1
  delayMatch33/1 -> HwModeRegister33/1
  delayMatch8/1 -> HwModeRegister25/1
  delayMatch22/1 -> HwModeRegister53/1
  delayMatch36/1 -> HwModeRegister17/1
  delayMatch12/1 -> HwModeRegister41/1
  delayMatch26/1 -> HwModeRegister55/1
  delayMatch40/1 -> HwModeRegister19/1
  Goto14/1 -> From/1
  Goto45/1 -> From34/1, From12/1, From1/1
  Goto6/1 -> From10/1
  Goto7/1 -> From11/1
  Goto46/1 -> From37/1, From2/1, From13/1
  Goto16/1 -> From14/1
  Goto11/1 -> From39/1, From31/1, From15/1
  Goto12/1 -> From54/1, From21/1, From16/1
  Goto13/1 -> From59/1, From22/1, From17/1
  Goto1/1 -> From57/1, From51/1, From50/1, From49/1, From18/1
  Goto8/1 -> From53/1, From20/1, From19/1
  Goto47/1 -> From4/1, From38/1, From23/1
  Goto42/1 -> From60/1, From29/1, From24/1
  Goto48/1 -> From5/1, From40/1, From25/1
  Goto43/1 -> From61/1, From32/1, From26/1
  Goto44/1 -> From62/1, From33/1, From27/1
  Goto21/1 -> From28/1
  Goto3/1 -> From7/1, From3/1
  Goto20/1 -> From30/1
  Goto41/1 -> From64/1, From43/1, From35/1
  Goto19/1 -> From36/1
  Goto9/1 -> From63/1, From52/1, From41/1
  Goto18/1 -> From42/1
  Goto10/1 -> From65/1, From55/1, From44/1
  Goto35/1 -> From45/1
  Goto49/1 -> From80/1, From56/1, From46/1
  Goto36/1 -> From47/1
  Goto/1 -> From48/1
  Goto15/1 -> From6/1
  Goto4/1 -> From8/1
  Goto5/1 -> From9/1
  Sum21_stage2/1 -> Sum21_stage3/1
  Gain_const/1 -> HwModeRegister56/1
  Gain1_const/1 -> HwModeRegister58/1
  Gain11_const/1 -> HwModeRegister60/1
  Gain13_const/1 -> HwModeRegister62/1
  Gain15_const/1 -> HwModeRegister64/1
  Gain18_const/1 -> HwModeRegister66/1
  Gain20_const/1 -> HwModeRegister68/1
  Gain22_const/1 -> HwModeRegister70/1
  Gain24_const/1 -> HwModeRegister72/1
  Gain25_const/1 -> HwModeRegister74/1
  Gain26_const/1 -> HwModeRegister76/1
  Gain27_const/1 -> HwModeRegister78/1
  Gain31_const/1 -> HwModeRegister80/1
  Gain32_const/1 -> HwModeRegister82/1
  Gain33_const/1 -> HwModeRegister84/1
  Gain34_const/1 -> HwModeRegister86/1
  Gain9_const/1 -> HwModeRegister88/1
  HEX3/2(Out2) -> delayMatch/1
  Logical Operator21/1 -> delayMatch1/1
  aPA_Save/1(MulResult) -> delayMatch2/1
  From56/1 -> delayMatch3/1
  Logical Operator13/1 -> delayMatch4/1
  bPA_Save/1(MulResult) -> delayMatch5/1
  From55/1 -> delayMatch6/1
  Logical Operator14/1 -> delayMatch7/1
  cPA_Save/1(MulResult) -> delayMatch8/1
  From52/1 -> delayMatch9/1
  From11/1 -> delayMatch10/1
  Logical Operator17/1 -> delayMatch11/1
  dPA_Save/1(MulResult) -> delayMatch12/1
  From19/1 -> delayMatch13/1
  From17/1 -> delayMatch14/1
  Logical Operator23/1 -> delayMatch15/1
  aPB_Save/1(MulResult) -> delayMatch16/1
  From46/1 -> delayMatch17/1
  Logical Operator19/1 -> delayMatch18/1
  bPB_Save/1(MulResult) -> delayMatch19/1
  From44/1 -> delayMatch20/1
  Logical Operator20/1 -> delayMatch21/1
  cPB_Save/1(MulResult) -> delayMatch22/1
  From41/1 -> delayMatch23/1
  Sum23/1 -> delayMatch24/1
  Logical Operator22/1 -> delayMatch25/1
  dPB_Save/1(MulResult) -> delayMatch26/1
  From20/1 -> delayMatch27/1
  From22/1 -> delayMatch28/1
  Logical Operator49/1 -> delayMatch29/1
  aPC_Save/1(MulResult) -> delayMatch30/1
  From80/1 -> delayMatch31/1
  Logical Operator41/1 -> delayMatch32/1
  bPC_Save/1(MulResult) -> delayMatch33/1
  From65/1 -> delayMatch34/1
  Logical Operator42/1 -> delayMatch35/1
  cPC_Save/1(MulResult) -> delayMatch36/1
  From63/1 -> delayMatch37/1
  From42/1 -> delayMatch38/1
  Logical Operator45/1 -> delayMatch39/1
  dPC_Save/1(MulResult) -> delayMatch40/1
  From53/1 -> delayMatch41/1
  From59/1 -> delayMatch42/1
  From49/1 -> delayMatch43/1
  From45/1 -> delayMatch44/1
  SW15/1 -> delayMatch45/1
  From50/1 -> delayMatch46/1
  From39/1 -> delayMatch47/1
  delayMatch66/1 -> Sample_Pulse/1
  From18/1 -> delayMatch49/1
  From51/1 -> delayMatch50/1
  From57/1 -> delayMatch51/1
  DAC Control/1("CLK ") -> delayMatch52/1
  DAC Control/2(Sync_n) -> delayMatch53/1
  DAC Control/3(Blank_n) -> delayMatch54/1
  HEX0/1(HEX0) -> delayMatch55/1
  HEX1/1(HEX1) -> delayMatch56/1
  HEX2/1(HEX2) -> delayMatch57/1
  HEX3/1(HEX3) -> delayMatch58/1
  Logical Operator8/1 -> delayMatch59/1, Subsystem11/1(In1)
  Logical Operator10/1 -> delayMatch60/1
  Logical Operator24/1 -> delayMatch61/1, Subsystem12/1(In1)
  Logical Operator18/1 -> delayMatch62/1
  Logical Operator51/1 -> delayMatch63/1, Subsystem13/1(In1)
  Logical Operator38/1 -> delayMatch64/1
  Multiport Switch1/1 -> delayMatch65/1
  Logical Operator27/1 -> delayMatch66/1, delayMatch48/1, Goto1/1, HDL Counter12/2
  Subsystem11/1(Out1) -> delayMatch67/1
  Subsystem12/1(Out1) -> delayMatch68/1
  Subsystem13/1(Out1) -> delayMatch69/1
  Logical Operator/1 -> Subsystem/Enable
  Unit Delay/1 -> Logical Operator/1
  Logical Operator1/1 -> Subsystem1/Enable
  Unit Delay1/1 -> Logical Operator1/1
  Logical Operator2/1 -> Subsystem2/Enable
  Unit Delay2/1 -> Logical Operator2/1
  Logical Operator7/1 -> Subsystem7/Enable
  Unit Delay7/1 -> Logical Operator7/1
  Logical Operator4/1 -> Subsystem4/Enable
  Unit Delay4/1 -> Logical Operator4/1
  Logical Operator5/1 -> Subsystem5/Enable
  Unit Delay5/1 -> Logical Operator5/1
  Logical Operator6/1 -> Subsystem6/Enable
  Unit Delay6/1 -> Logical Operator6/1
  HDL Counter12/1 -> Relational Operator2/1
  Relational Operator2/1 -> Logical Operator26/1
  Logical Operator26/1 -> Logical Operator27/1
  Logical Operator3/1 -> Subsystem3/Enable
  Unit Delay3/1 -> Logical Operator3/1
  Multiply/1 -> PipelineRegister/1
  HwModeRegister/1 -> Multiply/1
  HwModeRegister1/1 -> Multiply/2
  Multiply1/1 -> PipelineRegister1/1
  HwModeRegister2/1 -> Multiply1/1
  HwModeRegister3/1 -> Multiply1/2
  Multiply10/1 -> PipelineRegister2/1
  HwModeRegister4/1 -> Multiply10/1
  HwModeRegister5/1 -> Multiply10/2
  Multiply11/1 -> PipelineRegister3/1
  HwModeRegister6/1 -> Multiply11/1
  HwModeRegister7/1 -> Multiply11/2
  Multiply12/1 -> PipelineRegister4/1
  HwModeRegister8/1 -> Multiply12/1
  HwModeRegister9/1 -> Multiply12/2
  Multiply13/1 -> PipelineRegister5/1
  HwModeRegister10/1 -> Multiply13/1
  HwModeRegister11/1 -> Multiply13/2
  Multiply14/1 -> PipelineRegister6/1
  HwModeRegister12/1 -> Multiply14/1
  HwModeRegister13/1 -> Multiply14/2
  Multiply15/1 -> PipelineRegister7/1
  HwModeRegister14/1 -> Multiply15/1
  HwModeRegister15/1 -> Multiply15/2
  Multiply16/1 -> PipelineRegister8/1
  HwModeRegister16/1 -> Multiply16/1
  HwModeRegister17/1 -> Multiply16/2
  Multiply17/1 -> PipelineRegister9/1
  HwModeRegister18/1 -> Multiply17/1
  HwModeRegister19/1 -> Multiply17/2
  Multiply18/1 -> PipelineRegister10/1
  HwModeRegister20/1 -> Multiply18/1
  HwModeRegister21/1 -> Multiply18/2
  Multiply19/1 -> PipelineRegister11/1
  HwModeRegister22/1 -> Multiply19/1
  HwModeRegister23/1 -> Multiply19/2
  Multiply2/1 -> PipelineRegister12/1
  HwModeRegister24/1 -> Multiply2/1
  HwModeRegister25/1 -> Multiply2/2
  Multiply20/1 -> PipelineRegister13/1
  HwModeRegister26/1 -> Multiply20/1
  HwModeRegister27/1 -> Multiply20/2
  Multiply21/1 -> PipelineRegister14/1
  HwModeRegister28/1 -> Multiply21/1
  HwModeRegister29/1 -> Multiply21/2
  Multiply22/1 -> PipelineRegister15/1
  HwModeRegister30/1 -> Multiply22/1
  HwModeRegister31/1 -> Multiply22/2
  Multiply23/1 -> PipelineRegister16/1
  HwModeRegister32/1 -> Multiply23/1
  HwModeRegister33/1 -> Multiply23/2
  Multiply27/1 -> PipelineRegister17/1
  HwModeRegister34/1 -> Multiply27/1
  HwModeRegister35/1 -> Multiply27/2
  Multiply28/1 -> PipelineRegister18/1
  HwModeRegister36/1 -> Multiply28/1
  HwModeRegister37/1 -> Multiply28/2
  Multiply29/1 -> PipelineRegister19/1
  HwModeRegister38/1 -> Multiply29/1
  HwModeRegister39/1 -> Multiply29/2
  Multiply3/1 -> PipelineRegister20/1
  HwModeRegister40/1 -> Multiply3/1
  HwModeRegister41/1 -> Multiply3/2
  Multiply30/1 -> PipelineRegister21/1
  HwModeRegister42/1 -> Multiply30/1
  HwModeRegister43/1 -> Multiply30/2
  Multiply4/1 -> PipelineRegister22/1
  HwModeRegister44/1 -> Multiply4/1
  HwModeRegister45/1 -> Multiply4/2
  Multiply5/1 -> PipelineRegister23/1
  HwModeRegister46/1 -> Multiply5/1
  HwModeRegister47/1 -> Multiply5/2
  Multiply6/1 -> PipelineRegister24/1
  HwModeRegister48/1 -> Multiply6/1
  HwModeRegister49/1 -> Multiply6/2
  Multiply7/1 -> PipelineRegister25/1
  HwModeRegister50/1 -> Multiply7/1
  HwModeRegister51/1 -> Multiply7/2
  Multiply8/1 -> PipelineRegister26/1
  HwModeRegister52/1 -> Multiply8/1
  HwModeRegister53/1 -> Multiply8/2
  Multiply9/1 -> PipelineRegister27/1
  HwModeRegister54/1 -> Multiply9/1
  HwModeRegister55/1 -> Multiply9/2
  Gain/1 -> PipelineRegister28/1
  HwModeRegister56/1 -> Gain/1
  HwModeRegister57/1 -> Gain/2
  Gain1/1 -> PipelineRegister29/1
  HwModeRegister58/1 -> Gain1/1
  HwModeRegister59/1 -> Gain1/2
  Gain11/1 -> PipelineRegister30/1
  HwModeRegister60/1 -> Gain11/1
  HwModeRegister61/1 -> Gain11/2
  Gain13/1 -> PipelineRegister31/1
  HwModeRegister62/1 -> Gain13/1
  HwModeRegister63/1 -> Gain13/2
  Gain15/1 -> PipelineRegister32/1
  HwModeRegister64/1 -> Gain15/1
  HwModeRegister65/1 -> Gain15/2
  Gain18/1 -> PipelineRegister33/1
  HwModeRegister66/1 -> Gain18/1
  HwModeRegister67/1 -> Gain18/2
  Gain20/1 -> PipelineRegister34/1
  HwModeRegister68/1 -> Gain20/1
  HwModeRegister69/1 -> Gain20/2
  Gain22/1 -> PipelineRegister35/1
  HwModeRegister70/1 -> Gain22/1
  HwModeRegister71/1 -> Gain22/2
  Gain24/1 -> PipelineRegister36/1
  HwModeRegister72/1 -> Gain24/1
  HwModeRegister73/1 -> Gain24/2
  Gain25/1 -> PipelineRegister37/1
  HwModeRegister74/1 -> Gain25/1
  HwModeRegister75/1 -> Gain25/2
  Gain26/1 -> PipelineRegister38/1
  HwModeRegister76/1 -> Gain26/1
  HwModeRegister77/1 -> Gain26/2
  Gain27/1 -> PipelineRegister39/1
  HwModeRegister78/1 -> Gain27/1
  HwModeRegister79/1 -> Gain27/2
  Gain31/1 -> PipelineRegister40/1
  HwModeRegister80/1 -> Gain31/1
  HwModeRegister81/1 -> Gain31/2
  Gain32/1 -> PipelineRegister41/1
  HwModeRegister82/1 -> Gain32/1
  HwModeRegister83/1 -> Gain32/2
  Gain33/1 -> PipelineRegister42/1
  HwModeRegister84/1 -> Gain33/1
  HwModeRegister85/1 -> Gain33/2
  Gain34/1 -> PipelineRegister43/1
  HwModeRegister86/1 -> Gain34/1
  HwModeRegister87/1 -> Gain34/2
  Gain9/1 -> PipelineRegister44/1
  HwModeRegister88/1 -> Gain9/1
  HwModeRegister89/1 -> Gain9/2

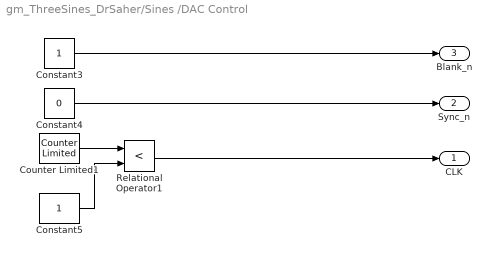
== system gm_ThreeSines_DrSaher/Sines /DAC Control ==
  Constant3 : Constant  OutDataTypeStr=boolean  SampleTime=ST
  Constant4 : Constant  Value=0  OutDataTypeStr=boolean  SampleTime=ST
  Constant5 : Constant  OutMax=[1]  OutDataTypeStr=uint32  SampleTime=ST
  Counter Limited1 : simulink/Sources/Counter Limited  uplimit=1  tsamp=ST
  Relational Operator1 : RelationalOperator  Operator=<  OutDataTypeStr=boolean  RndMeth=Simplest
  "CLK " : Outport  OutDataTypeStr=boolean
  Sync_n : Outport  Port=2
  Blank_n : Outport  Port=3
  wires:
  Constant3/1 -> Blank_n/1
  Constant4/1 -> Sync_n/1
  Constant5/1 -> Relational Operator1/2
  Counter Limited1/1 -> Relational Operator1/1
  Relational Operator1/1 -> "CLK "/1
